simulink library "NeuroMuscularLibrary"  (R2019b)
settings: Solver=ode45  StartTime=0.0  StopTime=10.0  RelTol=1e-3  EnableMultiTasking=on
values from neighbouring files (symbols this model uses):
  a_18_19 = 116    [Prosthesis3R60Params.m]
  a_18_21 = 34    [Prosthesis3R60Params.m]
  a_2_3 = 18    [Prosthesis3R60Params.m]
  angle_offset = 0    [Prosthesis3R60Params.m]
  ankle_height = 0.08    [BodyMechParams.m]
  c = 0.05    [BodyMechParams.m]
  c_jointstop = 0.3 / (pi/180)    (= 17.1887338539)    [BodyMechParams.m]
  c_stance_comp_a0 = 885.0653    [Prosthesis3R60Params.m]
  c_stance_comp_a1 = 2.1443    [Prosthesis3R60Params.m]
  cg14 = 1/2*L14    (= 0.0475)    [Prosthesis3R60Params.m]
  cg25 = (5.45/11.05)*L25    (= 0.0379527149321)    [Prosthesis3R60Params.m]
  cg3 = (3.6/10.4)*L3    (= 0.0306346153846)    [Prosthesis3R60Params.m]
  d_fBall = 0.1    [BodyMechParams.m]
  d_fHeel = 0.05    [BodyMechParams.m]
  deltaLegAngleThr = 8*pi/180    (= 0.13962634016)    [CMGParams.m]
  DeltaThRef = 2e-3    (= 0.002)    [BodyMechParams.m]
  dt_visual = 0.001    [Prosthesis3R60Params.m]
  eref = 0.04    [BodyMechParams.m]
  Fmax = 4000    [MuscleEnergyTest.m]
  FmaxGLU = 1500    [BodyMechParams.m]
  footBallToAnkleDist = 0.16    [BodyMechParams.m]
  footBallToCenterDist = footLength/2    (= 0.1)    [BodyMechParams.m]
  footBallToHeelDist = footLength    (= 0.2)    [BodyMechParams.m]
  footCenterToCGDist = 0.14 - footBallToCenterDist    (= 0.04)    [BodyMechParams.m]
  footInertia = 0.005    [BodyMechParams.m]
  footLength = 0.2    [BodyMechParams.m]
  footMass = 1.25    [BodyMechParams.m]
  FT = 20    [MuscleEnergyTest.m]
  FT_GLU = 47.6    [BodyMechParams.m]
  g = 9.80665    [BodyMechParams.m]
  groundTheta = [atan(diff(groundZ)./diff(groundX)), 0]    [generateGround.m]
  groundZ = groundZ * stepSize/(largestStep+eps)    [generateGround.m]
  hatCenterToCGDist = 0.35 - hatHipToCenterDistLen    (= -0.05)    [BodyMechParams.m]
  hatHipToCenterDistLen = hatLength/2    (= 0.4)    [BodyMechParams.m]
  hatInertia = 3    [BodyMechParams.m]
  hatLeftHipToCenterDistWidth = .15    (= 0.15)    [BodyMechParams.m]
  hatLength = 0.8    [BodyMechParams.m]
  hatMass = 53.5    [BodyMechParams.m]
  hatThickness = 0.2    [BodyMechParams.m]
  hatWidth = 0.4    [BodyMechParams.m]
  J1011 = (4130)*1e-9    (= 4.13e-06)    [Prosthesis3R60Params.m]
  J1415 = (1.18*1e5)*1e-9    (= 0.000118)    [Prosthesis3R60Params.m]
  J18192021 = (6.86*1e4)*1e-9    (= 6.86e-05)    [Prosthesis3R60Params.m]
  J2526 = (3.59*1e4)*1e-9    (= 3.59e-05)    [Prosthesis3R60Params.m]
  J3467 = (25.96*1e4)*1e-9    (= 0.0002596)    [Prosthesis3R60Params.m]
  K = 5    [BodyMechParams.m]
  k_gn = k_gn/2    (= 39226.6)    [BodyMechParams.m]
  k_gt = k_gt/2    (= 39226.6)    [BodyMechParams.m]
  k_pressure = hatMass * g / DeltaThRef    (= 262327.8875)    [BodyMechParams.m]
  k_stance = 130000    [Prosthesis3R60Params.m]
  k_swing = 18750    [Prosthesis3R60Params.m]
  L0_stance = 0.08925    [Prosthesis3R60Params.m]
  L0_swing = 0.0896    [Prosthesis3R60Params.m]
  L10 = 7.9*1e-3    (= 0.0079)    [Prosthesis3R60Params.m]
  L11 = 3.3*1e-3    (= 0.0033)    [Prosthesis3R60Params.m]
  L14 = 95*1e-3    (= 0.095)    [Prosthesis3R60Params.m]
  L15 = 8.2*1e-3    (= 0.0082)    [Prosthesis3R60Params.m]
  L18 = 25.1*1e-3    (= 0.0251)    [Prosthesis3R60Params.m]
  L19 = 17.7*1e-3    (= 0.0177)    [Prosthesis3R60Params.m]
  L20 = 26*1e-3    (= 0.026)    [Prosthesis3R60Params.m]
  L21 = 1.7*1e-3    (= 0.0017)    [Prosthesis3R60Params.m]
  L25 = 76.95*1e-3    (= 0.07695)    [Prosthesis3R60Params.m]
  L26 = 2.8*1e-3    (= 0.0028)    [Prosthesis3R60Params.m]
  L3 = 88.5*1e-3    (= 0.0885)    [Prosthesis3R60Params.m]
  L4 = 1.7*1e-3    (= 0.0017)    [Prosthesis3R60Params.m]
  L6 = 40.25*1e-3    (= 0.04025)    [Prosthesis3R60Params.m]
  L7 = 14.9*1e-3    (= 0.0149)    [Prosthesis3R60Params.m]
  leg_l = [(thighLength - ankle_height/2) (shankLength - ankle_height/2)]    [BodyMechParams.m]
  legAngleSpeedMax = 10    [CMGParams.m]
  lopt = 0.055    [MuscleEnergyTest.m]
  loptBFSH = 0.12    [BodyMechParams.m]
  loptGAS = 0.05    [BodyMechParams.m]
  loptGLU = 0.11    [BodyMechParams.m]
  loptHAB = 0.09    [BodyMechParams.m]
  loptHAD = 0.10    (= 0.1)    [BodyMechParams.m]
  loptHAM = 0.10    (= 0.1)    [BodyMechParams.m]
  loptHFL = 0.11    [BodyMechParams.m]
  loptRF = 0.08    [BodyMechParams.m]
  loptSOL = 0.04    [BodyMechParams.m]
  loptTA = 0.06    [BodyMechParams.m]
  loptVAS = 0.08    [BodyMechParams.m]
  lslack = 0.245    [MuscleEnergyTest.m]
  lslackBFSH = 0.10    (= 0.1)    [BodyMechParams.m]
  lslackGAS = 0.40    (= 0.4)    [BodyMechParams.m]
  lslackGLU = 0.13    [BodyMechParams.m]
  lslackHAB = 0.07    [BodyMechParams.m]
  lslackHAD = 0.18    [BodyMechParams.m]
  lslackHAM = 0.31    [BodyMechParams.m]
  lslackHFL = 0.10    (= 0.1)    [BodyMechParams.m]
  lslackRF = 0.35    [BodyMechParams.m]
  lslackSOL = 0.26    [BodyMechParams.m]
  lslackTA = 0.24    [BodyMechParams.m]
  lslackVAS = 0.23    [BodyMechParams.m]
  m1011 = 49.5*1e-3    (= 0.0495)    [Prosthesis3R60Params.m]
  m1415 = 123.8*1e-3    (= 0.1238)    [Prosthesis3R60Params.m]
  m18192021 = 196.6*1e-3    (= 0.1966)    [Prosthesis3R60Params.m]
  m2526 = 58.3*1e-3    (= 0.0583)    [Prosthesis3R60Params.m]
  m3467 = 253.3*1e-3    (= 0.2533)    [Prosthesis3R60Params.m]
  mu_slide = 0.8    [BodyMechParams.m]
  mu_stick = 0.9    [BodyMechParams.m]
  N = 1.5    [BodyMechParams.m]    (also in cmaes.m = size(x,1); mergeCompareEnergyCosts.m = {S.name})
  phiKneeUpLimit = 5*pi/180    (= 0.0872664625997)    [BodyMechParams.m]
  phimaxGASa = (100-90)*pi/180    (= 0.174532925199)    [BodyMechParams.m]
  phimaxGASk = (180-140)*pi/180    (= 0.698131700798)    [BodyMechParams.m]
  phimaxRFk = (180-165)*pi/180    (= 0.261799387799)    [BodyMechParams.m]
  phimaxSOL = (100-90)*pi/180    (= 0.174532925199)    [BodyMechParams.m]
  phimaxTA = (80-90)*pi/180    (= -0.174532925199)    [BodyMechParams.m]
  phimaxVAS = (180-165)*pi/180    (= 0.261799387799)    [BodyMechParams.m]
  phirefBFSH = (180-160)*pi/180    (= 0.349065850399)    [BodyMechParams.m]
  phirefGASa = (80-90)*pi/180    (= -0.174532925199)    [BodyMechParams.m]
  phirefGASk = (180-165)*pi/180    (= 0.261799387799)    [BodyMechParams.m]
  phirefGLU = (120-180)*pi/180    (= -1.0471975512)    [BodyMechParams.m]
  phirefHAB = 10*pi/180    (= 0.174532925199)    [BodyMechParams.m]
  phirefHAD = 15*pi/180    (= 0.261799387799)    [BodyMechParams.m]
  phirefHAMh = (150-180)*pi/180    (= -0.523598775598)    [BodyMechParams.m]
  phirefHAMk = (180-180)*pi/180    (= 0)    [BodyMechParams.m]
  phirefHFL = (160-180)*pi/180    (= -0.349065850399)    [BodyMechParams.m]
  phirefRFh = (170-180)*pi/180    (= -0.174532925199)    [BodyMechParams.m]
  phirefRFk = (180-125)*pi/180    (= 0.959931088597)    [BodyMechParams.m]
  phirefSOL = (90-90)*pi/180    (= 0)    [BodyMechParams.m]
  ... (+64 more)
undefined symbols (not defined in the file or in its folder): ankleBackDriveGain, ankleCJointstop, ankleDgain, ankleFilterPID, ankleFilterSEA, ankleGearEff, ankleGearRatio, ankleIgain, ankleInitialAngle, ankleInputMass, ankleIntCoulomb, ankleIntDamping, ankleIntStatic, ankleParallelSpringDamping, ankleParallelSpringOffset, ankleParallelSpringStiffness, anklePgain, anklePlantarLimit, ankleSEADamping, ankleSEAStiffness, ankleTendonMass, ankleWMaxJointstop, D12_F, D12_S, D12_T, D12z_T, D13_F, D1G_F, D1G_HAT, D1G_S, D1G_T, D1Gy_F, DeltaS, DeltaSGLU, DeltaSHFL, dryFrictionDamping, dryFrictionStiffness, dryFrictionVelThresh, footMassp, FourBarL1, FourBarL3, GainDphiHATGLUst, GainDphiHATHABst, GainDphiHATHADst, GainDphiHATHFLst, GainFGASst, GainFGLUst, GainFHABst, GainFHAMst, GainFSOLst, GainFSOLTAst, GainFVASst, GainGAS, GainGLU, GainGLUswing, GainHAM, GainHAMHFL ... (+194)
libraries: sm_lib x332, nesl_utility x156, simulink x33, dspswit3 x30, $bdroot x19, simulink_extras x7
(part 10 of 15)

== system NeuroMuscularLibrary/VAS Link ==
  note: VAS Attachment
  Knee angle [rad] : Inport
  Constant : Constant  Value=lslackVAS+loptVAS
  Constant1 : Constant  Value=phimaxVAS
  Constant2 : Constant  Value=phirefVAS
  Demux : Demux  Outputs=2
  Gain1 : Gain  Gain=rVASmax
  Gain3 : Gain  Gain=phiScaleVAS
  Gain4 : Gain  Gain=rhoVAS/phiScaleVAS
  Gain5 : Gain  Gain=phiScaleVAS
  Multiply : Gain  Gain=-1
  Mux : Mux  Inputs=2
  Sum1 : Sum  Inputs=-+
  Sum2 : Sum  Inputs=|+-
  Sum3 : Sum  Inputs=-+|
  Sum5 : Sum  Inputs=|++
  length change term : Trigonometry
  offset correction term : Trigonometry
  variable lever term : Trigonometry  Operator=cos
  lmtu [m] : Outport
  lever [m] : Outport  Port=2
  wires:
  Sum1/1 -> Mux/1
  Sum5/1 -> lmtu [m]/1
  offset correction term/1 -> Sum1/1
  Sum2/1 -> Gain5/1
  Constant1/1 -> Sum3/1, Sum2/2
  Constant/1 -> Sum5/1
  Gain3/1 -> variable lever term/1, length change term/1
  Gain1/1 -> Demux/1
  length change term/1 -> Sum1/2
  Constant2/1 -> Sum2/1
  Demux/1 -> Multiply/1
  Mux/1 -> Gain1/1
  Gain4/1 -> Sum5/2
  Demux/2 -> lever [m]/1
  variable lever term/1 -> Mux/2
  Sum3/1 -> Gain3/1
  Gain5/1 -> offset correction term/1
  Knee angle [rad]/1 -> Sum3/2
  Multiply/1 -> Gain4/1

== system NeuroMuscularLibrary/Velocity Sensor ==
  Mux : Mux  Inputs=3
  PS-Simulink Converter : nesl_utility/PS-Simulink Converter  PhysicalDomain=network_engine_domain  SubClassName=ps_output  LeftPortType=input  RightPortType=output  PseudoPeriodic=off  Frequencies=[]  Unit=m/s  AffineConversion=off
  PS-Simulink Converter1 : nesl_utility/PS-Simulink Converter  PhysicalDomain=network_engine_domain  SubClassName=ps_output  LeftPortType=input  RightPortType=output  PseudoPeriodic=off  Frequencies=[]  Unit=m/s  AffineConversion=off
  PS-Simulink Converter2 : nesl_utility/PS-Simulink Converter  PhysicalDomain=network_engine_domain  SubClassName=ps_output  LeftPortType=input  RightPortType=output  PseudoPeriodic=off  Frequencies=[]  Unit=m/s  AffineConversion=off
  Position Sensor : sm_lib/Frames and Transforms/Transform Sensor  MeasurementFrame=World  SenseAngle=off  SenseAxis=off  SenseAngle1=off  SenseAngle2=off  SenseAngle3=off  SenseQ=off  SenseR=off  SenseOmegaX=off  SenseOmegaY=off  SenseOmegaZ=off  SenseOmega1=off  SenseOmega2=off  SenseOmega3=off  SenseQDot=off  SenseRDot=off  SenseAlphaX=off  SenseAlphaY=off  SenseAlphaZ=off  SenseAlpha1=off  SenseAlpha2=off  SenseAlpha3=off  SenseQDDot=off  SenseRDDot=off  SenseX=off  SenseY=off  SenseZ=off  SenseRad=off  SenseAzim=off  SenseDist=off  SenseInc=off  SenseXDot=on  SenseYDot=on  SenseZDot=on  SenseRadDot=off  SenseAzimDot=off  SenseDistDot=off  SenseIncDot=off  SenseXDDot=off  SenseYDDot=off  SenseZDDot=off  SenseRadDDot=off  SenseAzimDDot=off  SenseDistDDot=off  SenseIncDDot=off
  World Frame : sm_lib/Frames and Transforms/World Frame
  Frame : PMIOPort  Side=Left
  Velocity : Outport
  wires:
  PS-Simulink Converter1/1 -> Mux/2
  PS-Simulink Converter/1 -> Mux/1
  Mux/1 -> Velocity/1
  PS-Simulink Converter2/1 -> Mux/3
  connections:
  Position Sensor/LConn1 -- World Frame/RConn1
  Position Sensor/RConn3 -- PS-Simulink Converter1/LConn1
  Position Sensor/RConn1 -- Frame/RConn1
  Position Sensor/RConn2 -- PS-Simulink Converter/LConn1
  Position Sensor/RConn4 -- PS-Simulink Converter2/LConn1

== system NeuroMuscularLibrary/c ==
  Velocity : Inport
  AND : Logic  Operator=OR  AllPortsSameDT=off  OutDataTypeStr=boolean
  Abs : Abs  ZeroCross=off
  Add3 : Sum
  Cast To Double : DataTypeConversion  OutDataTypeStr=double
  Constant1 : Constant  Value=a1
  Constant2 : Constant  Value=a0
  Constant3 : Constant  Value=0
  IsInf : RelationalOperator  Operator=isInf  OutDataTypeStr=boolean  ZeroCross=off  RndMeth=Simplest
  IsNaN : RelationalOperator  Operator=isNaN  OutDataTypeStr=boolean  ZeroCross=off  RndMeth=Simplest
  Product : Product  Inputs=/*
  Product1 : Product
  Switch : Switch  Criteria=u2 ~= 0  ZeroCross=off
  F_damper : Outport
  wires:
  Constant2/1 -> Add3/2
  Abs/1 -> Product/1
  Constant1/1 -> Product/2
  Product/1 -> Add3/1
  Product1/1 -> Switch/3, IsInf/1, IsNaN/1
  IsNaN/1 -> AND/1
  IsInf/1 -> AND/2
  AND/1 -> Cast To Double/1
  Cast To Double/1 -> Switch/2
  Constant3/1 -> Switch/1
  Switch/1 -> F_damper/1
  Velocity/1 -> Product1/1, Abs/1
  Add3/1 -> Product1/2  "c"

== system NeuroMuscularLibrary/Full Prosthesis/Ankle  Joint ==
  Torque on Ankle : Inport
  Ankle Joint : sm_lib/Joints/Revolute Joint  JointMode=Normal  SenseConstraintForce=off  SenseConstraintForceX=off  SenseConstraintForceY=off  SenseConstraintForceZ=off  SenseConstraintTorque=off  SenseConstraintTorqueX=off  SenseConstraintTorqueY=off  SenseConstraintTorqueZ=off  SenseTotalForce=off  SenseTotalForceX=off  SenseTotalForceY=off  SenseTotalForceZ=off  SenseTotalTorque=off  SenseTotalTorqueX=off  SenseTotalTorqueY=off  SenseTotalTorqueZ=off  CompositeWrenchDir=FollowerOnBase  CompositeWrenchFrame=BaseFrame  EquilibriumPosition=0  EquilibriumPositionUnits=deg  SpringStiffness=0  SpringStiffnessUnits=N*m/rad  DampingCoefficient=0  DampingCoefficientUnits=N*m/(rad/s)  TorqueActuationMode=InputTorque  MotionActuationMode=ComputedMotion  SensePosition=on  SenseVelocity=on  SenseAcceleration=off  SenseTorqueForce=off  SenseLowerLimitTorqueForce=off  SenseUpperLimitTorqueForce=off  LowerLimitSpecify=off  LowerLimitBound=-90  LowerLimitBoundUnits=deg  LowerLimitStiffness=1e4  LowerLimitStiffnessUnits=N*m/deg  LowerLimitDamping=10  LowerLimitDampingUnits=N*m/(deg/s)  LowerLimitTransitionRegionWidth=0.1  LowerLimitTransitionRegionWidthUnits=deg  UpperLimitSpecify=off  UpperLimitBound=90  UpperLimitBoundUnits=deg  UpperLimitStiffness=1e4  UpperLimitStiffnessUnits=N*m/deg  UpperLimitDamping=10  UpperLimitDampingUnits=N*m/(deg/s)  UpperLimitTransitionRegionWidth=0.1  UpperLimitTransitionRegionWidthUnits=deg  PositionTargetSpecify=on  PositionTargetPriority=Low  PositionTargetValue=0  PositionTargetValueUnits=rad  VelocityTargetSpecify=off  VelocityTargetPriority=High  VelocityTargetValue=0  VelocityTargetValueUnits=deg/s
  Ankle Plantarflexion Limit : Subsystem  mask{phiUpLimit=anklePlantarLimit, ext=-1, c_jointstop=ankleCJointstop, w_max_jointstop=ankleWMaxJointstop}
      mask prompts: phiUpLimit "Upper Limit [rad]"; ext "Extension values are positive or negative?"; c_jointstop "Stiffness"; w_max_jointstop "Max retraction speed"
      mask help:
      | This block implements a hard joint limit that will prevent the joint from extending past the specified upper limit.
      |
      | Used for the knee and hip joints.
  PS-Simulink Converter2 : nesl_utility/PS-Simulink Converter  PhysicalDomain=network_engine_domain  SubClassName=ps_output  LeftPortType=input  RightPortType=output  PseudoPeriodic=off  Frequencies=[]  Unit=rad  AffineConversion=off
  PS-Simulink Converter3 : nesl_utility/PS-Simulink Converter  PhysicalDomain=network_engine_domain  SubClassName=ps_output  LeftPortType=input  RightPortType=output  PseudoPeriodic=off  Frequencies=[]  Unit=rad/s  AffineConversion=off
  Simulink-PS Converter : nesl_utility/Simulink-PS Converter  PhysicalDomain=network_engine_domain  SubClassName=ps_input  LeftPortType=input  RightPortType=output  PseudoPeriodic=off  Frequencies=[]  NoiseDistribution=none  NoiseParameters=[]  Unit=N*m  AffineConversion=off  FilteringAndDerivatives=zero  SimscapeFilterOrder=1  InputFilterTimeConstant=0.001  UdotUserProvided=1
  Sum : Sum  Inputs=|++
  Ankle : PMIOPort  Side=Left
  Foot : PMIOPort  Port=2  Side=Right
  Ankle Angle : Outport
  Ankle Speed : Outport  Port=2
  Actual Torque : Outport  Port=3
  Ankle Stop Torque : Outport  Port=4
  wires:
  PS-Simulink Converter3/1 -> Ankle Speed/1, Ankle Plantarflexion Limit/2(dphi [rad/s])
  Sum/1 -> Actual Torque/1, Simulink-PS Converter/1
  Torque on Ankle/1 -> Sum/1
  PS-Simulink Converter2/1 -> Ankle Angle/1, Ankle Plantarflexion Limit/1(phi [rad])
  Ankle Plantarflexion Limit/1(M_stop [Nm]) -> Sum/2, Ankle Stop Torque/1
  connections:
  Ankle Joint/LConn2 -- Simulink-PS Converter/RConn1
  Ankle Joint/RConn2 -- PS-Simulink Converter2/LConn1
  Ankle Joint/RConn3 -- PS-Simulink Converter3/LConn1
  Ankle Joint/RConn1 -- Foot/RConn1
  Ankle Joint/LConn1 -- Ankle/RConn1

== system NeuroMuscularLibrary/Full Prosthesis/Ankle Input Joint ==
  Torque on Ankle Input : Inport
  Ankle Input Joint : sm_lib/Joints/Revolute Joint  JointMode=Normal  SenseConstraintForce=off  SenseConstraintForceX=off  SenseConstraintForceY=off  SenseConstraintForceZ=off  SenseConstraintTorque=off  SenseConstraintTorqueX=off  SenseConstraintTorqueY=off  SenseConstraintTorqueZ=off  SenseTotalForce=off  SenseTotalForceX=off  SenseTotalForceY=off  SenseTotalForceZ=off  SenseTotalTorque=off  SenseTotalTorqueX=off  SenseTotalTorqueY=off  SenseTotalTorqueZ=off  CompositeWrenchDir=FollowerOnBase  CompositeWrenchFrame=BaseFrame  EquilibriumPosition=0  EquilibriumPositionUnits=rad  SpringStiffness=0  SpringStiffnessUnits=N*m/deg  DampingCoefficient=0  DampingCoefficientUnits=N*m/(deg/s)  TorqueActuationMode=InputTorque  MotionActuationMode=ComputedMotion  SensePosition=on  SenseVelocity=on  SenseAcceleration=on  SenseTorqueForce=off  SenseLowerLimitTorqueForce=off  SenseUpperLimitTorqueForce=off  LowerLimitSpecify=off  LowerLimitBound=-90  LowerLimitBoundUnits=deg  LowerLimitStiffness=1e4  LowerLimitStiffnessUnits=N*m/deg  LowerLimitDamping=10  LowerLimitDampingUnits=N*m/(deg/s)  LowerLimitTransitionRegionWidth=0.1  LowerLimitTransitionRegionWidthUnits=deg  UpperLimitSpecify=off  UpperLimitBound=90  UpperLimitBoundUnits=deg  UpperLimitStiffness=1e4  UpperLimitStiffnessUnits=N*m/deg  UpperLimitDamping=10  UpperLimitDampingUnits=N*m/(deg/s)  UpperLimitTransitionRegionWidth=0.1  UpperLimitTransitionRegionWidthUnits=deg  PositionTargetSpecify=on  PositionTargetPriority=High  PositionTargetValue=ankleInitialAngle  PositionTargetValueUnits=rad  VelocityTargetSpecify=off  VelocityTargetPriority=High  VelocityTargetValue=0  VelocityTargetValueUnits=deg/s
  PS-Simulink Converter1 : nesl_utility/PS-Simulink Converter  PhysicalDomain=network_engine_domain  SubClassName=ps_output  LeftPortType=input  RightPortType=output  PseudoPeriodic=off  Frequencies=[]  Unit=rad/s^2  AffineConversion=off
  PS-Simulink Converter2 : nesl_utility/PS-Simulink Converter  PhysicalDomain=network_engine_domain  SubClassName=ps_output  LeftPortType=input  RightPortType=output  PseudoPeriodic=off  Frequencies=[]  Unit=rad  AffineConversion=off
  PS-Simulink Converter3 : nesl_utility/PS-Simulink Converter  PhysicalDomain=network_engine_domain  SubClassName=ps_output  LeftPortType=input  RightPortType=output  PseudoPeriodic=off  Frequencies=[]  Unit=rad/s  AffineConversion=off
  Rigid Transform : sm_lib/Frames and Transforms/Rigid Transform  TranslationMethod=None  TranslationStandardOffset=0  TranslationLengthUnit=m  TranslationStandardAxis=+Z  TranslationCartesianOffset=[0 0 0]  TranslationROffset=0  TranslationROffsetUnits=m  TranslationZOffset=0  TranslationZOffsetUnits=m  TranslationThetaOffset=0  TranslationThetaOffsetUnits=deg  RotationMethod=StandardAxis  RotationAngleUnits=deg  RotationStandardAxis=+Z  RotationAngle=180  RotationArbitraryAxis=[0 0 1]  FollAlignAxisA=+X  BaseAlignAxisA=+Y  FollAlignAxisB=+Y  BaseAlignAxisB=+Z  RotationSequenceAxes=FollowerAxes  RotationSequence=XYX  RotationSequenceAngles=[0 0 0]  RotationSequenceAnglesUnits=deg  RotationMatrix=[1 0 0; 0 1 0; 0 0 1]
  Simulink-PS Converter : nesl_utility/Simulink-PS Converter  PhysicalDomain=network_engine_domain  SubClassName=ps_input  LeftPortType=input  RightPortType=output  PseudoPeriodic=off  Frequencies=[]  NoiseDistribution=none  NoiseParameters=[]  Unit=N*m  AffineConversion=off  FilteringAndDerivatives=zero  SimscapeFilterOrder=1  InputFilterTimeConstant=0.001  UdotUserProvided=1
  Ankle Stator : PMIOPort  Side=Right
  Ankle Input : PMIOPort  Port=2  Side=Left
  Ankle Input Angle : Outport
  Ankle Input Speed : Outport  Port=2
  Ankle Input Accel : Outport  Port=3
  wires:
  PS-Simulink Converter2/1 -> Ankle Input Angle/1
  PS-Simulink Converter3/1 -> Ankle Input Speed/1
  PS-Simulink Converter1/1 -> Ankle Input Accel/1
  Torque on Ankle Input/1 -> Simulink-PS Converter/1
  connections:
  Ankle Input Joint/RConn1 -- Ankle Input/RConn1
  Ankle Input Joint/RConn3 -- PS-Simulink Converter3/LConn1
  Ankle Input Joint/RConn2 -- PS-Simulink Converter2/LConn1
  Ankle Input Joint/LConn2 -- Simulink-PS Converter/RConn1
  Ankle Input Joint/RConn4 -- PS-Simulink Converter1/LConn1
  Ankle Input Joint/LConn1 -- Rigid Transform/RConn1
  Rigid Transform/LConn1 -- Ankle Stator/RConn1

== system NeuroMuscularLibrary/Full Prosthesis/Ankle Input Link ==
  CG : sm_lib/Frames and Transforms/Reference Frame
  Shank : sm_lib/Body Elements/File Solid  ExtGeomFileName=ankleInputLink.STL  UnitType=Custom  ExtGeomFileUnits=mm  StepReaderType=HEX  ExportEntireGeometry=off  InertiaType=Custom  Mass=ankleInputMass  MassUnits=g  CenterOfMass=ankleInputCG  CenterOfMassUnits=mm  MomentsOfInertia=ankleInputMomentOfInertia  MomentsOfInertiaUnits=g*cm^2  ProductsOfInertia=ankleInputProductOfInertia  ProductsOfInertiaUnits=g*cm^2  BasedOnType=Density  Density=1000  DensityUnits=kg/(m^3)  DoExposeReferenceFrame=on  SerializedFrames=<Frames/>  GraphicType=FromGeometry  MarkerShape=Sphere  MarkerSize=10  MarkerSizeUnits=m  GraphicVisPropType=SimpleVisualProperties  GraphicDiffuseColor=[0.5 0.5 0.5]  GraphicSpecularColor=[0.5 0.5 0.5 1.0]  GraphicAmbientColor=[0.15 0.15 0.15 1.0]  GraphicEmissiveColor=[0.0 0.0 0.0 1.0]  GraphicShininess=75  GraphicOpacity=1.0
  To CG : sm_lib/Frames and Transforms/Rigid Transform  TranslationMethod=Cartesian  TranslationStandardOffset=1.5  TranslationLengthUnit=mm  TranslationStandardAxis=-Z  TranslationCartesianOffset=ankleInputCG  TranslationROffset=0  TranslationROffsetUnits=m  TranslationZOffset=0  TranslationZOffsetUnits=m  TranslationThetaOffset=0  TranslationThetaOffsetUnits=deg  RotationMethod=None  RotationAngleUnits=deg  RotationStandardAxis=+Z  RotationAngle=0  RotationArbitraryAxis=[0 0 1]  FollAlignAxisA=+X  BaseAlignAxisA=+Y  FollAlignAxisB=+Y  BaseAlignAxisB=+Z  RotationSequenceAxes=FollowerAxes  RotationSequence=XYX  RotationSequenceAngles=[0 0 0]  RotationSequenceAnglesUnits=deg  RotationMatrix=[1 0 0; 0 1 0; 0 0 1]
  To Tendon : sm_lib/Frames and Transforms/Rigid Transform  TranslationMethod=Cartesian  TranslationStandardOffset=445.61  TranslationLengthUnit=mm  TranslationStandardAxis=-Y  TranslationCartesianOffset=[80, 0, 2]  TranslationROffset=0  TranslationROffsetUnits=m  TranslationZOffset=0  TranslationZOffsetUnits=m  TranslationThetaOffset=0  TranslationThetaOffsetUnits=deg  RotationMethod=None  RotationAngleUnits=deg  RotationStandardAxis=+Z  RotationAngle=0  RotationArbitraryAxis=[0 0 1]  FollAlignAxisA=+X  BaseAlignAxisA=+Y  FollAlignAxisB=+Y  BaseAlignAxisB=+Z  RotationSequenceAxes=FollowerAxes  RotationSequence=XYX  RotationSequenceAngles=[0 0 0]  RotationSequenceAnglesUnits=deg  RotationMatrix=[1 0 0; 0 1 0; 0 0 1]
  " Ankle Input Joint" : PMIOPort  Side=Right
  Tendon : PMIOPort  Port=2  Side=Left
  connections:
  Tendon/RConn1 -- To Tendon/RConn1
  CG/RConn1 -- To CG/RConn1
  To Tendon/LConn1 -- " Ankle Input Joint"/RConn1 -- To CG/LConn1 -- Shank/RConn1

== system NeuroMuscularLibrary/Full Prosthesis/Ankle Motor ==
  Voltage : Inport
  Net Motor Torque : Inport  Port=2
  Load Speed : Inport  Port=3
  Ankle Motor Axis : sm_lib/Joints/Revolute Joint  JointMode=Normal  SenseConstraintForce=off  SenseConstraintForceX=off  SenseConstraintForceY=off  SenseConstraintForceZ=off  SenseConstraintTorque=off  SenseConstraintTorqueX=off  SenseConstraintTorqueY=off  SenseConstraintTorqueZ=off  SenseTotalForce=off  SenseTotalForceX=off  SenseTotalForceY=off  SenseTotalForceZ=off  SenseTotalTorque=off  SenseTotalTorqueX=off  SenseTotalTorqueY=off  SenseTotalTorqueZ=off  CompositeWrenchDir=FollowerOnBase  CompositeWrenchFrame=BaseFrame  EquilibriumPosition=0  EquilibriumPositionUnits=deg  SpringStiffness=0  SpringStiffnessUnits=N*m/deg  DampingCoefficient=0  DampingCoefficientUnits=N*m/(deg/s)  TorqueActuationMode=InputTorque  MotionActuationMode=ComputedMotion  SensePosition=on  SenseVelocity=on  SenseAcceleration=off  SenseTorqueForce=off  SenseLowerLimitTorqueForce=off  SenseUpperLimitTorqueForce=off  LowerLimitSpecify=off  LowerLimitBound=-90  LowerLimitBoundUnits=deg  LowerLimitStiffness=1e4  LowerLimitStiffnessUnits=N*m/deg  LowerLimitDamping=10  LowerLimitDampingUnits=N*m/(deg/s)  LowerLimitTransitionRegionWidth=0.1  LowerLimitTransitionRegionWidthUnits=deg  UpperLimitSpecify=off  UpperLimitBound=90  UpperLimitBoundUnits=deg  UpperLimitStiffness=1e4  UpperLimitStiffnessUnits=N*m/deg  UpperLimitDamping=10  UpperLimitDampingUnits=N*m/(deg/s)  UpperLimitTransitionRegionWidth=0.1  UpperLimitTransitionRegionWidthUnits=deg  PositionTargetSpecify=on  PositionTargetPriority=High  PositionTargetValue=-ankleInitialAngle*ankleGearRatio  PositionTargetValueUnits=rad  VelocityTargetSpecify=off  VelocityTargetPriority=High  VelocityTargetValue=0  VelocityTargetValueUnits=deg/s
  Friction : Subsystem  Commented=on  mask{Fs=ankleIntStatic, Fc=ankleIntCoulomb, sigma0=dryFrictionStiffness, sigma1=dryFrictionDamping, v_s=dryFrictionVelThresh, Fv=ankleIntDamping}
      mask prompts: Fs "Static Friction"; Fc "Colulomb Friction"; sigma0 "Dry Friction Stiffness"; sigma1 "Dry Friction Damping"; v_s "Velocity Threshold"; Fv "Viscous Friction"
  Gain : Gain  Gain=-1
  Motor Dynamics : Subsystem
  PS-Simulink Converter : nesl_utility/PS-Simulink Converter  PhysicalDomain=network_engine_domain  SubClassName=ps_output  LeftPortType=input  RightPortType=output  PseudoPeriodic=off  Frequencies=[]  Unit=rad  AffineConversion=off
  PS-Simulink Converter1 : nesl_utility/PS-Simulink Converter  PhysicalDomain=network_engine_domain  SubClassName=ps_output  LeftPortType=input  RightPortType=output  PseudoPeriodic=off  Frequencies=[]  Unit=rad/s  AffineConversion=off
  Scope : Scope  NumInputPorts=2
  Simulink-PS Converter : nesl_utility/Simulink-PS Converter  PhysicalDomain=network_engine_domain  SubClassName=ps_input  LeftPortType=input  RightPortType=output  PseudoPeriodic=off  Frequencies=[]  NoiseDistribution=none  NoiseParameters=[]  Unit=N*m  AffineConversion=off  FilteringAndDerivatives=zero  SimscapeFilterOrder=1  InputFilterTimeConstant=0.001  UdotUserProvided=1
  Sum : Sum  Inputs=+|+
  Ankle Stator : PMIOPort  Side=Right
  Ankle Rotor : PMIOPort  Port=2  Side=Left
  Motor Torque : Outport
  Motor Angle : Outport  Port=2
  Motor Speed : Outport  Port=3
  wires:
  Friction/1(Friction Force) -> Sum/2, Scope/2
  Voltage/1 -> Motor Dynamics/1(Voltage)
  PS-Simulink Converter/1 -> Motor Angle/1
  Net Motor Torque/1 -> Simulink-PS Converter/1
  PS-Simulink Converter1/1 -> Motor Dynamics/2(Speed), Motor Speed/1
  Motor Dynamics/1(Torque) -> Sum/1
  Sum/1 -> Motor Torque/1
  Load Speed/1 -> Gain/1
  Gain/1 -> Friction/1(Velocity), Scope/1
  connections:
  Ankle Motor Axis/LConn1 -- Ankle Stator/RConn1
  Ankle Motor Axis/RConn2 -- PS-Simulink Converter/LConn1
  Ankle Motor Axis/RConn3 -- PS-Simulink Converter1/LConn1
  Ankle Motor Axis/LConn2 -- Simulink-PS Converter/RConn1
  Ankle Motor Axis/RConn1 -- Ankle Rotor/RConn1

== system NeuroMuscularLibrary/Full Prosthesis/Ankle Motor Rotor ==
  CG : sm_lib/Frames and Transforms/Reference Frame
  Knee Rotor1 : sm_lib/Body Elements/File Solid  ExtGeomFileName=motorRotor.STL  UnitType=Custom  ExtGeomFileUnits=mm  StepReaderType=HEX  ExportEntireGeometry=off  InertiaType=Custom  Mass=motorRotorMass  MassUnits=g  CenterOfMass=motorRotorCG  CenterOfMassUnits=mm  MomentsOfInertia=motorRotorMomentOfInertia  MomentsOfInertiaUnits=g*cm^2  ProductsOfInertia=motorRotorProductOfInertia  ProductsOfInertiaUnits=g*cm^2  BasedOnType=Density  Density=1000  DensityUnits=kg/(m^3)  DoExposeReferenceFrame=on  SerializedFrames=<Frames/>  GraphicType=FromGeometry  MarkerShape=Sphere  MarkerSize=10  MarkerSizeUnits=m  GraphicVisPropType=SimpleVisualProperties  GraphicDiffuseColor=[0.5 0.5 0.5]  GraphicSpecularColor=[0.5 0.5 0.5 1.0]  GraphicAmbientColor=[0.15 0.15 0.15 1.0]  GraphicEmissiveColor=[0.0 0.0 0.0 1.0]  GraphicShininess=75  GraphicOpacity=1.0
  Rigid Transform : sm_lib/Frames and Transforms/Rigid Transform  TranslationMethod=StandardAxis  TranslationStandardOffset=4.5  TranslationLengthUnit=mm  TranslationStandardAxis=+Z  TranslationCartesianOffset=[0 0 0]  TranslationROffset=0  TranslationROffsetUnits=m  TranslationZOffset=0  TranslationZOffsetUnits=m  TranslationThetaOffset=0  TranslationThetaOffsetUnits=deg  RotationMethod=None  RotationAngleUnits=deg  RotationStandardAxis=+Z  RotationAngle=0  RotationArbitraryAxis=[0 0 1]  FollAlignAxisA=+X  BaseAlignAxisA=+Y  FollAlignAxisB=+Y  BaseAlignAxisB=+Z  RotationSequenceAxes=FollowerAxes  RotationSequence=XYX  RotationSequenceAngles=[0 0 0]  RotationSequenceAnglesUnits=deg  RotationMatrix=[1 0 0; 0 1 0; 0 0 1]
  ToCG : sm_lib/Frames and Transforms/Rigid Transform  TranslationMethod=Cartesian  TranslationStandardOffset=0  TranslationLengthUnit=mm  TranslationStandardAxis=+Z  TranslationCartesianOffset=motorRotorCG  TranslationROffset=0  TranslationROffsetUnits=m  TranslationZOffset=0  TranslationZOffsetUnits=m  TranslationThetaOffset=0  TranslationThetaOffsetUnits=deg  RotationMethod=None  RotationAngleUnits=deg  RotationStandardAxis=+Z  RotationAngle=0  RotationArbitraryAxis=[0 0 1]  FollAlignAxisA=+X  BaseAlignAxisA=+Y  FollAlignAxisB=+Y  BaseAlignAxisB=+Z  RotationSequenceAxes=FollowerAxes  RotationSequence=XYX  RotationSequenceAngles=[0 0 0]  RotationSequenceAnglesUnits=deg  RotationMatrix=[1 0 0; 0 1 0; 0 0 1]
  Conn1 : PMIOPort  Side=Right
  connections:
  CG/RConn1 -- ToCG/RConn1
  ToCG/LConn1 -- Knee Rotor1/RConn1 -- Rigid Transform/RConn1
  Conn1/RConn1 -- Rigid Transform/LConn1

== system NeuroMuscularLibrary/Full Prosthesis/Ankle Parallel Spring ==
  Ankle Angle : Inport
  Ankle Speed : Inport  Port=2
  Add : Sum
  Bias : Bias  Bias=-ankleParallelSpringOffset
  Parallel Spring Stiffness : Gain  Gain=-ankleParallelSpringStiffness
  Parallel Spring Damping : Gain  Gain=-ankleParallelSpringDamping
  Saturation1 : Saturate  UpperLimit=0  LowerLimit=-inf  ZeroCross=off
  Saturation2 : Saturate  UpperLimit=0  LowerLimit=-inf  ZeroCross=off
  Parallel Spring Torque : Outport
  wires:
  Add/1 -> Parallel Spring Torque/1
  Ankle Speed/1 -> Parallel Spring Damping/1
  Parallel Spring Stiffness/1 -> Saturation2/1
  Parallel Spring Damping/1 -> Saturation1/1
  Bias/1 -> Parallel Spring Stiffness/1
  Ankle Angle/1 -> Bias/1
  Saturation1/1 -> Add/2
  Saturation2/1 -> Add/1

== system NeuroMuscularLibrary/Full Prosthesis/Ankle SEA Control ==
  Motor Speed : Inport
  Load Acceleration : Inport  Port=2
  Measured Torque : Inport  Port=3
  Desired Ankle Torque : Inport  Port=4
  Parallel Spring Torque : Inport  Port=5
  Ankle Input Angle : Inport  Port=6
  Tendon Angle : Inport  Port=7
  Ankle Angle : Inport  Port=8
  4 bar ratio : Subsystem
  Divide : Product  Inputs=*/
  Feed Forward : Subsystem
  PID Controller : simulink/Continuous/PID Controller  Controller=PD  Form=Parallel  TimeDomain=Continuous-time  SampleTime=-1  IntegratorMethod=Forward Euler  FilterMethod=Forward Euler  ControllerParametersSource=internal  P=anklePgain  I=ankleIgain  D=ankleDgain  UseFilter=on  N=ankleFilterPID  TunerSelectOption=Transfer Function Based (PID Tuner App)  InitialConditionSource=internal  InitialConditionForIntegrator=0  InitialConditionForFilter=0  DifferentiatorICPrevScaledInput=0  ExternalReset=none  TrackingMode=off  Kt=1  LimitOutput=off  UpperSaturationLimit=inf  LowerSaturationLimit=-inf  LinearizeAsGain=on  AntiWindupMode=none  Kb=1  POutMin=[]  POutMax=[]  IOutMin=[]  IOutMax=[]  DOutMin=[]  DOutMax=[]  NOutMin=[]  NOutMax=[]  SumOutMin=[]  SumOutMax=[]  SaturationOutMin=[]  SaturationOutMax=[]  PParamMin=[]  PParamMax=[]  IParamMin=[]  IParamMax=[]  DParamMin=[]  DParamMax=[]  NParamMin=[]  NParamMax=[]  KbParamMin=[]  KbParamMax=[]  KtParamMin=[]  KtParamMax=[]  KbOutMin=[]  KbOutMax=[]  KtOutMin=[]  KtOutMax=[]  IntegratorOutMin=[]  IntegratorOutMax=[]  FilterOutMin=[]  FilterOutMax=[]  SumI1OutMin=[]  SumI1OutMax=[]  SumI2OutMin=[]  SumI2OutMax=[]  SumI3OutMin=[]  SumI3OutMax=[]  SumI4OutMin=[]  SumI4OutMax=[]  SumDOutMin=[]  SumDOutMax=[]  DifferentiatorOutMin=[]  DifferentiatorOutMax=[]  FilterDiffOutCoefMin=[]  FilterDiffOutCoefMax=[]  ReciprocalOutMin=[]  ReciprocalOutMax=[]  SumDenOutMin=[]  SumDenOutMax=[]  SumNumOutMin=[]  SumNumOutMax=[]  DivideOutMin=[]  DivideOutMax=[]  IntegratorContinuousStateAttributes=''  IntegratorStateMustResolveToSignalObject=off  IntegratorRTWStateStorageClass=Auto  FilterContinuousStateAttributes=''  FilterStateMustResolveToSignalObject=off  FilterRTWStateStorageClass=Auto  ParallelPVariant=InternalParameters  IdealPVariant=Disabled  IVariant=Disabled  DVariant=InternalParameters  IntegratorVariant=Disabled  SatVariant=Disabled  AWVariant=Disabled  PCopyVariant=Disabled  TRVariant=Disabled  FdbkBlocksVariant=Forward  IdealPFdbkVariant=Disabled  SatFdbkVariant=Disabled  DerivativeFilterVariant=ContFilter  NVariant=InternalParameters  NCopyVariant=Disabled  FilterICVariant=InternalICsFilter  IntegratorICVariant=Disabled  ExternalResetVariant=Disabled  TRSumVariant=Passthrough  SumFdbkVariant=Disabled  SumVariant=Sum_PD
  Saturation1 : Saturate  UpperLimit=motorMaxVoltage  LowerLimit=-motorMaxVoltage  ZeroCross=off
  Sum : Sum  Inputs=|+-
  Sum1 : Sum  Inputs=+-|
  Sum2 : Sum  Inputs=|+-
  Motor Voltage : Outport
  Desired Actuator Torque : Outport  Port=2
  wires:
  Divide/1 -> Sum/1, Feed Forward/3(Desired Actuator Torque), Desired Actuator Torque/1  "Desired Actuator"
  Sum2/1 -> Divide/1
  Saturation1/1 -> Motor Voltage/1
  Sum1/1 -> Saturation1/1
  Load Acceleration/1 -> Feed Forward/2(Load Acceleration)
  Ankle Input Angle/1 -> 4 bar ratio/1(Ankle Input Angle)
  Tendon Angle/1 -> 4 bar ratio/2(Tendon Angle)
  Ankle Angle/1 -> 4 bar ratio/3(Ankle Angle)
  Measured Torque/1 -> Sum/2
  Sum/1 -> PID Controller/1
  4 bar ratio/1(ratio) -> Divide/2
  Motor Speed/1 -> Feed Forward/1(Motor Speed)
  Feed Forward/1(Computed Motor Voltage) -> Sum1/1
  Desired Ankle Torque/1 -> Sum2/1
  Parallel Spring Torque/1 -> Sum2/2
  PID Controller/1 -> Sum1/2

== system NeuroMuscularLibrary/Full Prosthesis/Ankle Tendon ==
  CG : sm_lib/Frames and Transforms/Reference Frame
  PS-Simulink Converter : nesl_utility/PS-Simulink Converter  PhysicalDomain=network_engine_domain  SubClassName=ps_output  LeftPortType=input  RightPortType=output  PseudoPeriodic=off  Frequencies=[]  Unit=1  AffineConversion=off
  Revolute Joint : sm_lib/Joints/Revolute Joint  JointMode=Normal  SenseConstraintForce=off  SenseConstraintForceX=off  SenseConstraintForceY=off  SenseConstraintForceZ=off  SenseConstraintTorque=off  SenseConstraintTorqueX=off  SenseConstraintTorqueY=off  SenseConstraintTorqueZ=off  SenseTotalForce=off  SenseTotalForceX=off  SenseTotalForceY=off  SenseTotalForceZ=off  SenseTotalTorque=off  SenseTotalTorqueX=off  SenseTotalTorqueY=off  SenseTotalTorqueZ=off  CompositeWrenchDir=FollowerOnBase  CompositeWrenchFrame=BaseFrame  EquilibriumPosition=0  EquilibriumPositionUnits=deg  SpringStiffness=0  SpringStiffnessUnits=N*m/deg  DampingCoefficient=0  DampingCoefficientUnits=N*m/(deg/s)  TorqueActuationMode=NoTorque  MotionActuationMode=ComputedMotion  SensePosition=on  SenseVelocity=off  SenseAcceleration=off  SenseTorqueForce=off  SenseLowerLimitTorqueForce=off  SenseUpperLimitTorqueForce=off  LowerLimitSpecify=off  LowerLimitBound=-90  LowerLimitBoundUnits=deg  LowerLimitStiffness=1e4  LowerLimitStiffnessUnits=N*m/deg  LowerLimitDamping=10  LowerLimitDampingUnits=N*m/(deg/s)  LowerLimitTransitionRegionWidth=0.1  LowerLimitTransitionRegionWidthUnits=deg  UpperLimitSpecify=off  UpperLimitBound=90  UpperLimitBoundUnits=deg  UpperLimitStiffness=1e4  UpperLimitStiffnessUnits=N*m/deg  UpperLimitDamping=10  UpperLimitDampingUnits=N*m/(deg/s)  UpperLimitTransitionRegionWidth=0.1  UpperLimitTransitionRegionWidthUnits=deg  PositionTargetSpecify=off  PositionTargetPriority=High  PositionTargetValue=0  PositionTargetValueUnits=deg  VelocityTargetSpecify=off  VelocityTargetPriority=High  VelocityTargetValue=0  VelocityTargetValueUnits=deg/s
  Revolute Joint1 : sm_lib/Joints/Revolute Joint  JointMode=Normal  SenseConstraintForce=off  SenseConstraintForceX=off  SenseConstraintForceY=off  SenseConstraintForceZ=off  SenseConstraintTorque=off  SenseConstraintTorqueX=off  SenseConstraintTorqueY=off  SenseConstraintTorqueZ=off  SenseTotalForce=off  SenseTotalForceX=off  SenseTotalForceY=off  SenseTotalForceZ=off  SenseTotalTorque=off  SenseTotalTorqueX=off  SenseTotalTorqueY=off  SenseTotalTorqueZ=off  CompositeWrenchDir=FollowerOnBase  CompositeWrenchFrame=BaseFrame  EquilibriumPosition=0  EquilibriumPositionUnits=deg  SpringStiffness=0  SpringStiffnessUnits=N*m/deg  DampingCoefficient=0  DampingCoefficientUnits=N*m/(deg/s)  TorqueActuationMode=NoTorque  MotionActuationMode=ComputedMotion  SensePosition=off  SenseVelocity=off  SenseAcceleration=off  SenseTorqueForce=off  SenseLowerLimitTorqueForce=off  SenseUpperLimitTorqueForce=off  LowerLimitSpecify=off  LowerLimitBound=-90  LowerLimitBoundUnits=deg  LowerLimitStiffness=1e4  LowerLimitStiffnessUnits=N*m/deg  LowerLimitDamping=10  LowerLimitDampingUnits=N*m/(deg/s)  LowerLimitTransitionRegionWidth=0.1  LowerLimitTransitionRegionWidthUnits=deg  UpperLimitSpecify=off  UpperLimitBound=90  UpperLimitBoundUnits=deg  UpperLimitStiffness=1e4  UpperLimitStiffnessUnits=N*m/deg  UpperLimitDamping=10  UpperLimitDampingUnits=N*m/(deg/s)  UpperLimitTransitionRegionWidth=0.1  UpperLimitTransitionRegionWidthUnits=deg  PositionTargetSpecify=off  PositionTargetPriority=High  PositionTargetValue=0  PositionTargetValueUnits=deg  VelocityTargetSpecify=off  VelocityTargetPriority=High  VelocityTargetValue=0  VelocityTargetValueUnits=deg/s
  Shank : sm_lib/Body Elements/File Solid  ExtGeomFileName=ankleTendon.STL  UnitType=Custom  ExtGeomFileUnits=mm  StepReaderType=HEX  ExportEntireGeometry=off  InertiaType=Custom  Mass=ankleTendonMass  MassUnits=g  CenterOfMass=ankleTendonCG  CenterOfMassUnits=mm  MomentsOfInertia=ankleTendonMomentOfInertia  MomentsOfInertiaUnits=g*cm^2  ProductsOfInertia=ankleTendonProductOfInertia  ProductsOfInertiaUnits=g*cm^2  BasedOnType=Density  Density=1000  DensityUnits=kg/(m^3)  DoExposeReferenceFrame=on  SerializedFrames=<Frames/>  GraphicType=FromGeometry  MarkerShape=Sphere  MarkerSize=10  MarkerSizeUnits=m  GraphicVisPropType=SimpleVisualProperties  GraphicDiffuseColor=[0.5 0.5 0.5]  GraphicSpecularColor=[0.5 0.5 0.5 1.0]  GraphicAmbientColor=[0.15 0.15 0.15 1.0]  GraphicEmissiveColor=[0.0 0.0 0.0 1.0]  GraphicShininess=75  GraphicOpacity=1.0
  To CG : sm_lib/Frames and Transforms/Rigid Transform  TranslationMethod=Cartesian  TranslationStandardOffset=1.5  TranslationLengthUnit=mm  TranslationStandardAxis=-Z  TranslationCartesianOffset=ankleTendonCG  TranslationROffset=0  TranslationROffsetUnits=m  TranslationZOffset=0  TranslationZOffsetUnits=m  TranslationThetaOffset=0  TranslationThetaOffsetUnits=deg  RotationMethod=None  RotationAngleUnits=deg  RotationStandardAxis=+Z  RotationAngle=0  RotationArbitraryAxis=[0 0 1]  FollAlignAxisA=+X  BaseAlignAxisA=+Y  FollAlignAxisB=+Y  BaseAlignAxisB=+Z  RotationSequenceAxes=FollowerAxes  RotationSequence=XYX  RotationSequenceAngles=[0 0 0]  RotationSequenceAnglesUnits=deg  RotationMatrix=[1 0 0; 0 1 0; 0 0 1]
  To Foot : sm_lib/Frames and Transforms/Rigid Transform  TranslationMethod=Cartesian  TranslationStandardOffset=445.61  TranslationLengthUnit=mm  TranslationStandardAxis=-Y  TranslationCartesianOffset=[0, -328.8, 0]  TranslationROffset=0  TranslationROffsetUnits=m  TranslationZOffset=0  TranslationZOffsetUnits=m  TranslationThetaOffset=0  TranslationThetaOffsetUnits=deg  RotationMethod=None  RotationAngleUnits=deg  RotationStandardAxis=+Z  RotationAngle=0  RotationArbitraryAxis=[0 0 1]  FollAlignAxisA=+X  BaseAlignAxisA=+Y  FollAlignAxisB=+Y  BaseAlignAxisB=+Z  RotationSequenceAxes=FollowerAxes  RotationSequence=XYX  RotationSequenceAngles=[0 0 0]  RotationSequenceAnglesUnits=deg  RotationMatrix=[1 0 0; 0 1 0; 0 0 1]
  " Ankle Input Joint" : PMIOPort  Side=Left
  Foot : PMIOPort  Port=2  Side=Right
  Angle : Outport
  wires:
  PS-Simulink Converter/1 -> Angle/1
  connections:
  CG/RConn1 -- To CG/RConn1
  To Foot/LConn1 -- Revolute Joint/RConn1 -- To CG/LConn1 -- Shank/RConn1
  Revolute Joint/LConn1 -- " Ankle Input Joint"/RConn1
  Revolute Joint1/LConn1 -- To Foot/RConn1
  Foot/RConn1 -- Revolute Joint1/RConn1
  Revolute Joint/RConn2 -- PS-Simulink Converter/LConn1

== system NeuroMuscularLibrary/Full Prosthesis/Foot ==
  CG : sm_lib/Frames and Transforms/Reference Frame
  Shank : sm_lib/Body Elements/File Solid  ExtGeomFileName=foot.STL  UnitType=Custom  ExtGeomFileUnits=mm  StepReaderType=HEX  ExportEntireGeometry=off  InertiaType=Custom  Mass=footMassp  MassUnits=g  CenterOfMass=footCG  CenterOfMassUnits=mm  MomentsOfInertia=footMomentOfInertia  MomentsOfInertiaUnits=g*cm^2  ProductsOfInertia=footProductOfInertia  ProductsOfInertiaUnits=g*cm^2  BasedOnType=Density  Density=1000  DensityUnits=kg/(m^3)  DoExposeReferenceFrame=on  SerializedFrames=<Frames/>  GraphicType=FromGeometry  MarkerShape=Sphere  MarkerSize=10  MarkerSizeUnits=m  GraphicVisPropType=SimpleVisualProperties  GraphicDiffuseColor=[0.5 0.5 0.5]  GraphicSpecularColor=[0.5 0.5 0.5 1.0]  GraphicAmbientColor=[0.15 0.15 0.15 1.0]  GraphicEmissiveColor=[0.0 0.0 0.0 1.0]  GraphicShininess=75  GraphicOpacity=1.0
  To Ball : sm_lib/Frames and Transforms/Rigid Transform  TranslationMethod=Cartesian  TranslationStandardOffset=445.61  TranslationLengthUnit=mm  TranslationStandardAxis=-Y  TranslationCartesianOffset=[165, -63, 0]  TranslationROffset=0  TranslationROffsetUnits=m  TranslationZOffset=0  TranslationZOffsetUnits=m  TranslationThetaOffset=0  TranslationThetaOffsetUnits=deg  RotationMethod=None  RotationAngleUnits=deg  RotationStandardAxis=+Z  RotationAngle=0  RotationArbitraryAxis=[0 0 1]  FollAlignAxisA=+X  BaseAlignAxisA=+Y  FollAlignAxisB=+Y  BaseAlignAxisB=+Z  RotationSequenceAxes=FollowerAxes  RotationSequence=XYX  RotationSequenceAngles=[0 0 0]  RotationSequenceAnglesUnits=deg  RotationMatrix=[1 0 0; 0 1 0; 0 0 1]
  To CG : sm_lib/Frames and Transforms/Rigid Transform  TranslationMethod=Cartesian  TranslationStandardOffset=1.5  TranslationLengthUnit=mm  TranslationStandardAxis=-Z  TranslationCartesianOffset=footCG  TranslationROffset=0  TranslationROffsetUnits=m  TranslationZOffset=0  TranslationZOffsetUnits=m  TranslationThetaOffset=0  TranslationThetaOffsetUnits=deg  RotationMethod=None  RotationAngleUnits=deg  RotationStandardAxis=+Z  RotationAngle=0  RotationArbitraryAxis=[0 0 1]  FollAlignAxisA=+X  BaseAlignAxisA=+Y  FollAlignAxisB=+Y  BaseAlignAxisB=+Z  RotationSequenceAxes=FollowerAxes  RotationSequence=XYX  RotationSequenceAngles=[0 0 0]  RotationSequenceAnglesUnits=deg  RotationMatrix=[1 0 0; 0 1 0; 0 0 1]
  To Heel : sm_lib/Frames and Transforms/Rigid Transform  TranslationMethod=Cartesian  TranslationStandardOffset=445.61  TranslationLengthUnit=mm  TranslationStandardAxis=-Y  TranslationCartesianOffset=[-60, -63, 0]  TranslationROffset=0  TranslationROffsetUnits=m  TranslationZOffset=0  TranslationZOffsetUnits=m  TranslationThetaOffset=0  TranslationThetaOffsetUnits=deg  RotationMethod=None  RotationAngleUnits=deg  RotationStandardAxis=+Z  RotationAngle=0  RotationArbitraryAxis=[0 0 1]  FollAlignAxisA=+X  BaseAlignAxisA=+Y  FollAlignAxisB=+Y  BaseAlignAxisB=+Z  RotationSequenceAxes=FollowerAxes  RotationSequence=XYX  RotationSequenceAngles=[0 0 0]  RotationSequenceAnglesUnits=deg  RotationMatrix=[1 0 0; 0 1 0; 0 0 1]
  To Tendon : sm_lib/Frames and Transforms/Rigid Transform  TranslationMethod=Cartesian  TranslationStandardOffset=445.61  TranslationLengthUnit=mm  TranslationStandardAxis=-Y  TranslationCartesianOffset=[-81, -16.3, 0]  TranslationROffset=0  TranslationROffsetUnits=m  TranslationZOffset=0  TranslationZOffsetUnits=m  TranslationThetaOffset=0  TranslationThetaOffsetUnits=deg  RotationMethod=None  RotationAngleUnits=deg  RotationStandardAxis=+Z  RotationAngle=0  RotationArbitraryAxis=[0 0 1]  FollAlignAxisA=+X  BaseAlignAxisA=+Y  FollAlignAxisB=+Y  BaseAlignAxisB=+Z  RotationSequenceAxes=FollowerAxes  RotationSequence=XYX  RotationSequenceAngles=[0 0 0]  RotationSequenceAnglesUnits=deg  RotationMatrix=[1 0 0; 0 1 0; 0 0 1]
  " Ankle Input Joint" : PMIOPort  Side=Right
  Tendon Bearing : PMIOPort  Port=2  Side=Left
  Ball : PMIOPort  Port=3  Side=Left
  Heel : PMIOPort  Port=4  Side=Right
  connections:
  Tendon Bearing/RConn1 -- To Tendon/RConn1
  CG/RConn1 -- To CG/RConn1
  To Tendon/LConn1 -- " Ankle Input Joint"/RConn1 -- Shank/RConn1 -- To CG/LConn1 -- To Heel/LConn1 -- To Ball/LConn1
  Ball/RConn1 -- To Ball/RConn1
  Heel/RConn1 -- To Heel/RConn1

== system NeuroMuscularLibrary/Full Prosthesis/Harmonic Drive// Series Elastic Actuator ==
  Motor Speed : Inport
  Motor Angle : Inport  Port=2
  Motor Torque : Inport  Port=3
  Load Angle : Inport  Port=4
  Load Speed : Inport  Port=5
  Add : Sum
  Damping : Gain  Gain=kneeSEADamping
  Gain : Gain  Gain=-1
  Mux : Mux  Inputs=2
  Ratio1 : Gain  Gain=1/kneeGearRatio
  Ratio2 : Gain  Gain=1/kneeGearRatio
  Ratio3 : Gain  Gain=1/kneeGearRatio
  Ratio4 : Gain  Gain=1/kneeGearEff
  Scope : Scope
  Stiffness : Gain  Gain=kneeSEAStiffness
  Sum : Sum  Inputs=|++
  Sum1 : Sum  Inputs=|++
  Sum2 : Sum  Inputs=++|
  Torque on Motor : Outport
  " Torque on Load" : Outport  Port=2
  wires:
  Mux/1 -> Scope/1
  Load Speed/1 -> Sum2/2
  Ratio3/1 -> Sum2/1
  Motor Torque/1 -> Sum1/2
  Ratio2/1 -> Ratio4/1
  Load Angle/1 -> Sum/1
  Add/1 -> Gain/1  "External Torque"
  Ratio1/1 -> Sum/2
  Sum1/1 -> Torque on Motor/1
  Stiffness/1 -> Add/2, Mux/1
  Sum/1 -> Stiffness/1
  Damping/1 -> Add/1, Mux/2
  Sum2/1 -> Damping/1
  Motor Speed/1 -> Ratio3/1
  Motor Angle/1 -> Ratio1/1
  Ratio4/1 -> Sum1/1
  Gain/1 -> " Torque on Load"/1, Ratio2/1

== system NeuroMuscularLibrary/Full Prosthesis/Harmonic Drive// Series Elastic Actuator1 ==
  Motor Speed : Inport
  Motor Angle : Inport  Port=2
  Motor Torque : Inport  Port=3
  Load Angle : Inport  Port=4
  Load Speed : Inport  Port=5
  Add : Sum
  Damping : Gain  Gain=ankleSEADamping
  Gain : Gain  Gain=-1
  Ratio1 : Gain  Gain=1/ankleGearRatio
  Ratio2 : Gain  Gain=1/ankleGearRatio
  Ratio3 : Gain  Gain=1/ankleGearRatio
  Ratio4 : Gain  Gain=1/ankleGearEff
  Stiffness : Gain  Gain=ankleSEAStiffness
  Sum : Sum  Inputs=|++
  Sum1 : Sum  Inputs=|++
  Sum2 : Sum  Inputs=++|
  Torque on Motor : Outport
  Torque on Load : Outport  Port=2
  wires:
  Gain/1 -> Torque on Load/1, Ratio2/1
  Load Speed/1 -> Sum2/2
  Ratio3/1 -> Sum2/1
  Motor Torque/1 -> Sum1/2
  Ratio2/1 -> Ratio4/1
  Load Angle/1 -> Sum/1
  Add/1 -> Gain/1  "External Torque"
  Ratio1/1 -> Sum/2
  Sum1/1 -> Torque on Motor/1
  Stiffness/1 -> Add/2
  Sum/1 -> Stiffness/1
  Damping/1 -> Add/1
  Sum2/1 -> Damping/1
  Motor Speed/1 -> Ratio3/1
  Motor Angle/1 -> Ratio1/1
  Ratio4/1 -> Sum1/1
